simulink library "CTRL_DSI_PedalRecalc"  (R2022a)
settings: Solver=VariableStepAuto  StartTime=0.0  StopTime=10.0  RelTol=1e-3
settings Model: Creator=blatak  LastModifiedBy=blatak

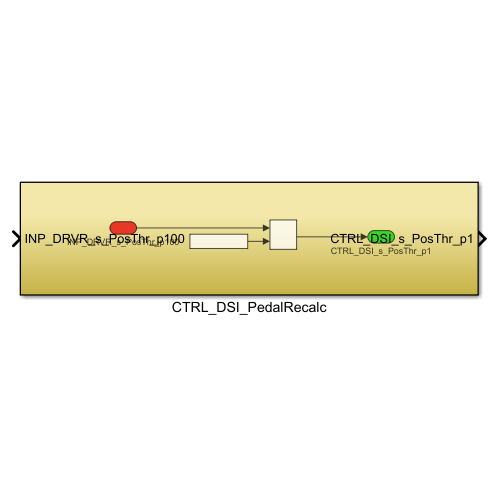
[thumbnail: Simulink's stored preview of the top-level diagram]
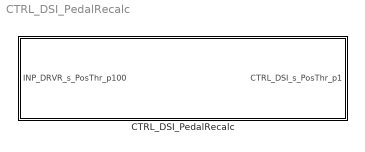
== system CTRL_DSI_PedalRecalc ==
  CTRL_DSI_PedalRecalc : Subsystem

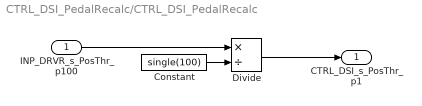
== system CTRL_DSI_PedalRecalc/CTRL_DSI_PedalRecalc ==
  INP_DRVR_s_PosThr_p100 : Inport
  Constant : Constant  Value=single(100)
  Divide : Product  Inputs=*/  RndMeth=Zero  SaturateOnIntegerOverflow=on
  CTRL_DSI_s_PosThr_p1 : Outport
  wires:
  Divide/1 -> CTRL_DSI_s_PosThr_p1/1
  INP_DRVR_s_PosThr_p100/1 -> Divide/1
  Constant/1 -> Divide/2
